simulink model "example4_pp_sim"  (R2020a)
settings: Solver=VariableStepAuto  StartTime=0.0  StopTime=10.0  RelTol=1e-3
values from neighbouring files (symbols this model uses):
  A = [0 1;2 3]    [example4_pp.m]
  B = [0;2]    [example4_pp.m]
  C = [1 0]    [example4_pp.m]    (also in example6_dcmotor.m = K_lqr * append(tf(1,[1 0]),1,1))
  K = acker(A,B,p)    [example4_pp.m]    (also in example6_dcmotor.m = 5)
  X_ini = [10; 10]    [example4_pp.m]
settings Model: Creator=Mook  LastModifiedBy=Mook

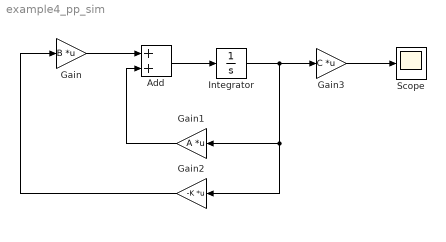
== system example4_pp_sim ==
  Add : Sum
  Gain : Gain  Gain=B  Multiplication=Matrix(K*u)
  Gain1 : Gain  Gain=A  Multiplication=Matrix(K*u)
  Gain2 : Gain  Gain=-K  Multiplication=Matrix(K*u)
  Gain3 : Gain  Gain=C  Multiplication=Matrix(K*u)
  Integrator : Integrator  InitialCondition=X_ini
  Scope : Scope
  wires:
  Gain/1 -> Add/1
  Add/1 -> Integrator/1
  Integrator/1 -> Gain2/1, Gain1/1, Gain3/1
  Gain3/1 -> Scope/1
  Gain1/1 -> Add/2
  Gain2/1 -> Gain/1
